simulink model "updatedModel"  (R2019a)
settings: Solver=FixedStepAuto  StartTime=0.0  StopTime=10  FixedStep=0.001  RelTol=1e-3
settings Model: Creator=houte  LastModifiedBy=coeng

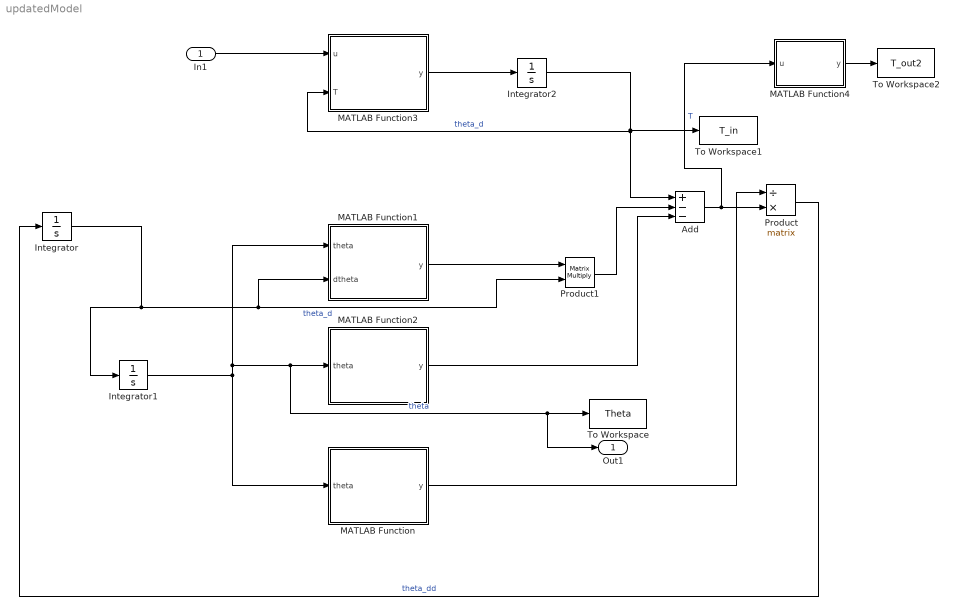
== system updatedModel ==
  In1 : Inport
  Add : Sum  Inputs=+--
  Integrator : Integrator  InitialCondition=[0; 0]
  Integrator1 : Integrator  InitialCondition=firstLocation'
  Integrator2 : Integrator  InitialCondition=[0; 0]
  MATLAB Function : MATLAB Function  TreatAsAtomicUnit=on
  MATLAB Function1 : MATLAB Function  TreatAsAtomicUnit=on
  MATLAB Function2 : MATLAB Function  TreatAsAtomicUnit=on
  MATLAB Function3 : MATLAB Function  TreatAsAtomicUnit=on
  MATLAB Function4 : MATLAB Function  TreatAsAtomicUnit=on
  Product : Product  Inputs=/*  Multiplication=Matrix(*)
  Product1 : Product  Multiplication=Matrix(*)
  To Workspace : ToWorkspace  VariableName=Theta  SaveFormat=Timeseries  SampleTime=-1
  To Workspace1 : ToWorkspace  VariableName=T_in  SaveFormat=Timeseries  SampleTime=-1
  To Workspace2 : ToWorkspace  VariableName=T_out2  SaveFormat=Timeseries  SampleTime=-1
  Out1 : Outport
  wires:
  Integrator/1 -> Product1/2, MATLAB Function1/2(dtheta), Integrator1/1  "theta_d"
  Integrator1/1 -> MATLAB Function1/1(theta), Out1/1, To Workspace/1, MATLAB Function2/1(theta), MATLAB Function/1(theta)  "theta"
  Add/1 -> MATLAB Function4/1(u), Product/2  "T"
  MATLAB Function1/1(y) -> Product1/1
  MATLAB Function3/1(y) -> Integrator2/1
  MATLAB Function2/1(y) -> Add/3
  MATLAB Function/1(y) -> Product/1
  Product/1 -> Integrator/1  "theta_dd"
  Integrator2/1 -> To Workspace1/1, MATLAB Function3/2(T), Add/1  "theta_d"
  Product1/1 -> Add/2
  MATLAB Function4/1(y) -> To Workspace2/1
  In1/1 -> MATLAB Function3/1(u)

== matlab function updatedModel/MATLAB Function1 ==
  data: theta input; y output; dtheta input; Parameters parameter
function y = C(theta, dtheta, Parameters)
    theta1 = theta(1);
    theta2 = theta(2);
    dtheta1 = dtheta(1);
    dtheta2 = dtheta(2);


y = [Parameters.b1 - Parameters.P3*dtheta2*sin(theta2), -Parameters.P3*(dtheta1+dtheta2)*sin(theta2);
    Parameters.P3*dtheta1*sin(theta2), Parameters.b2];

== matlab function updatedModel/MATLAB Function ==
  data: theta input; y output; Parameters parameter
function y = M(theta, Parameters)
theta1 = theta(1);
theta2 = theta(2);

y = [Parameters.P1 + Parameters.P2 + 2*Parameters.P3*cos(theta2), Parameters.P2 + Parameters.P3 * cos(theta2);
     Parameters.P2 + Parameters.P3*cos(theta2), Parameters.P2];

== matlab function updatedModel/MATLAB Function2 ==
  data: theta input; y output; Parameters parameter
function y = G(theta, Parameters)
    theta1 = theta(1);
    theta2 = theta(2);

y = [-Parameters.g1*sin(theta1) - Parameters.g2*sin(theta1+theta2);
     -Parameters.g2*sin(theta1+theta2)];

== matlab function updatedModel/MATLAB Function3 ==
  data: u input; y output; Parameters parameter; T input
function y = T(u, Parameters, T)
    % T = km*u - Te*dTe;
    %dTe = (km*u-T)/Te
    dTe = (Parameters.km*u-T(1))/Parameters.Te;
y = [dTe; 0];

== matlab function updatedModel/MATLAB Function4 ==
  data: u input; y output
function y = fcn(u)

y = u;
